simulink model "RobotControl"  (R2016a)
settings: Solver=FixedStepDiscrete  StartTime=0.0  StopTime=16  FixedStep=0.005  RelTol=1e-3
values from neighbouring files (symbols this model uses):
  BACKWARD = 2    [ControlInit.m]
  BUSY = 4    [ControlInit.m]
  CCW = 4    [ControlInit.m]
  CLEANED = 2    [ControlInit.m]
  CW = 3    [ControlInit.m]
  EMPTY = 3    [ControlInit.m]
  FORWARD = 1    [ControlInit.m]
  GTSP = 25    [ControlInit.m]
  initX = uint8((ROOM_SIDE_SIZE/2) - 1)    [ControlInit.m]
  initY = initX    [ControlInit.m]
  LEFT_BUSY_RIGHT_BUSY = 9    [ControlInit.m]
  LEFT_BUSY_RIGHT_CLEANED = 14    [ControlInit.m]
  LEFT_BUSY_RIGHT_EMPTY = 7    [ControlInit.m]
  LEFT_CLEANED_RIGHT_BUSY = 13    [ControlInit.m]
  LEFT_CLEANED_RIGHT_CLEANED = 12    [ControlInit.m]
  LEFT_CLEANED_RIGHT_EMPTY = 10    [ControlInit.m]
  LEFT_EMPTY_RIGHT_BUSY = 8    [ControlInit.m]
  LEFT_EMPTY_RIGHT_CLEANED = 11    [ControlInit.m]
  LEFT_EMPTY_RIGHT_EMPTY = 15    [ControlInit.m]
  map = uint8(ones(ROOM_SIDE_SIZE , ROOM_SIDE_SIZE)*UNCOVERED)    [ControlInit.m]
  MOVE_TURN_LEFT = 20    [ControlInit.m]
  MOVE_TURN_RIGHT = 21    [ControlInit.m]
  MOVE_U_TURN = 24    [ControlInit.m]
  MOVE_U_TURN_LEFT = 23    [ControlInit.m]
  MOVE_U_TURN_RIGHT = 22    [ControlInit.m]
  ROB_EAST = 0    [ControlInit.m]
  ROB_ERRVAL = 5    [ControlInit.m]
  ROB_NONE = 400    [ControlInit.m]
  ROB_NORTH = 270    [ControlInit.m]
  ROB_SOUTH = 90    [ControlInit.m]
  ROB_WEST = 180    [ControlInit.m]
  ROOM_SIDE_SIZE = 20    [ControlInit.m]
  STOP = 5    [ControlInit.m]
  UNCOVERED = 1    [ControlInit.m]
  ZIGZAG = 26    [ControlInit.m]
undefined symbols (not defined in the file or in its folder): COMH, Compass_Handler, MovementHandler, MOVH, POSH, positionHandler, ROB_LENG, ROTH, Routines, SAMPLE_TIME
libraries: simulink x2, SCAN x1, MAPH x1, MOTH x1
(part 1 of 2)
settings Model: Creator=oelkawok  LastModifiedBy=oelkawok
settings DataIOCC: SaveOutput=off  SaveTime=off

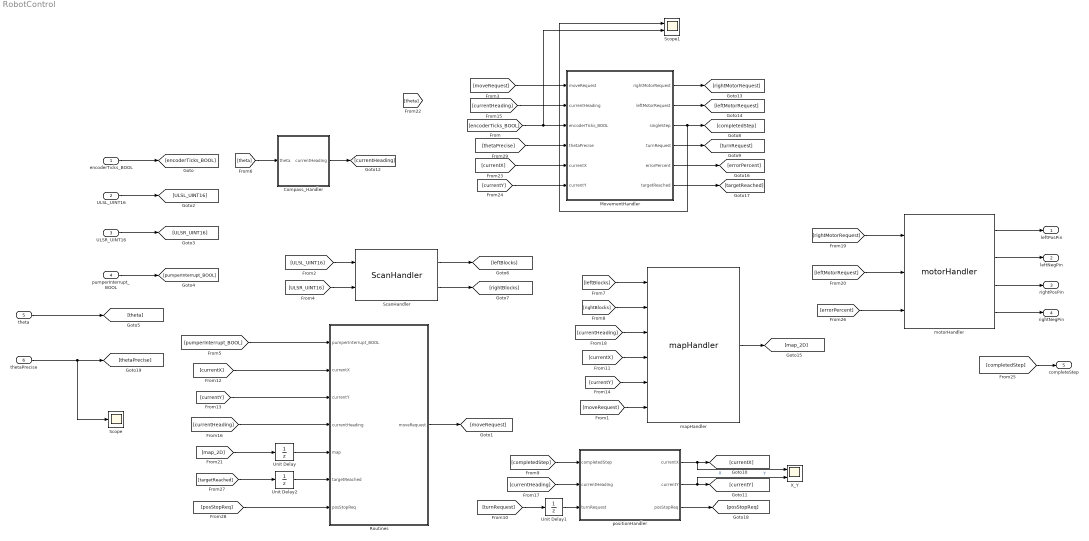
== system RobotControl ==
  encoderTicks_BOOL : Inport  OutDataTypeStr=boolean  PortDimensions=1
  ULSL_UINT16 : Inport  Port=2  PortDimensions=1
  ULSR_UINT16 : Inport  Port=3  PortDimensions=1
  pumperInterrupt_BOOL : Inport  Port=4  OutDataTypeStr=boolean  PortDimensions=1
  theta : Inport  Port=5  OutDataTypeStr=int16  PortDimensions=1
  thetaPrecise : Inport  Port=6  OutDataTypeStr=uint16  PortDimensions=1
  Compass_Handler : Subsystem  AncestorBlock=COMH/Compass_Handler
  MovementHandler : Subsystem  AncestorBlock=MOVH/MovementHandler
  Routines : Subsystem  AncestorBlock=ROTH/Routines
  ScanHandler : SCAN/ScanHandler
  Scope : Scope
  Scope1 : Scope  NumInputPorts=2
  Unit Delay : UnitDelay  InitialCondition=map  SampleTime=-1
      settings: AttributesFormatString=%<InitialCondition>
  Unit Delay1 : UnitDelay  InitialCondition=STOP  SampleTime=-1
      settings: AttributesFormatString=%<InitialCondition>
  Unit Delay2 : UnitDelay  SampleTime=-1
  X_Y : Scope  NumInputPorts=2
  mapHandler : MAPH/mapHandler
  motorHandler : MOTH/motorHandler
  positionHandler : Subsystem  AncestorBlock=POSH/positionHandler
  leftPosPin : Outport  OutDataTypeStr=double  PortDimensions=1
  leftNegPin : Outport  Port=2  OutDataTypeStr=double  PortDimensions=1
  rightPosPin : Outport  Port=3  OutDataTypeStr=double  PortDimensions=1
  rightNegPin : Outport  Port=4  OutDataTypeStr=double  PortDimensions=1
  completeStep : Outport  Port=5  PortDimensions=1
  wires:
  [moveRequest] -> MovementHandler/1(moveRequest)
  [encoderTicks_BOOL] -> MovementHandler/3(encoderTicks_BOOL), Scope1/2
  encoderTicks_BOOL/1 -> [encoderTicks_BOOL]
  ULSL_UINT16/1 -> [ULSL_UINT16]
  [ULSL_UINT16] -> ScanHandler/1
  ULSR_UINT16/1 -> [ULSR_UINT16]
  [ULSR_UINT16] -> ScanHandler/2
  pumperInterrupt_BOOL/1 -> [pumperInterrupt_BOOL]
  [pumperInterrupt_BOOL] -> Routines/1(pumperInterrupt_BOOL)
  Routines/1(moveRequest) -> [moveRequest]
  [moveRequest] -> mapHandler/6
  [theta] -> Compass_Handler/1(theta)
  ScanHandler/1 -> [leftBlocks]
  [leftBlocks] -> mapHandler/1
  ScanHandler/2 -> [rightBlocks]
  [rightBlocks] -> mapHandler/2
  MovementHandler/3(singleStep) -> Scope1/1, [completedStep]
  [completedStep] -> positionHandler/1(completedStep)
  MovementHandler/4(turnRequest) -> [turnRequest]
  [turnRequest] -> Unit Delay1/1
  positionHandler/1(currentX) -> X_Y/1, [currentX]  "X"
  [currentX] -> mapHandler/4
  [currentX] -> Routines/2(currentX)
  positionHandler/2(currentY) -> X_Y/2, [currentY]  "Y"
  [currentY] -> Routines/3(currentY)
  [currentY] -> mapHandler/5
  Compass_Handler/1(currentHeading) -> [currentHeading]
  [currentHeading] -> MovementHandler/2(currentHeading)
  [currentHeading] -> Routines/4(currentHeading)
  [currentHeading] -> positionHandler/2(currentHeading)
  [currentHeading] -> mapHandler/3
  [rightMotorRequest] -> motorHandler/1
  [leftMotorRequest] -> motorHandler/2
  MovementHandler/2(leftMotorRequest) -> [leftMotorRequest]
  MovementHandler/1(rightMotorRequest) -> [rightMotorRequest]
  motorHandler/4 -> rightNegPin/1
  motorHandler/2 -> leftNegPin/1
  motorHandler/3 -> rightPosPin/1
  motorHandler/1 -> leftPosPin/1
  mapHandler/1 -> [map_2D]
  [map_2D] -> Unit Delay/1
  Unit Delay/1 -> Routines/5(map)
  Unit Delay1/1 -> positionHandler/3(turnRequest)
  [currentX] -> MovementHandler/5(currentX)
  [currentY] -> MovementHandler/6(currentY)
  [completedStep] -> completeStep/1
  [errorPercent] -> motorHandler/3
  MovementHandler/5(errorPercent) -> [errorPercent]
  MovementHandler/6(targetReached) -> [targetReached]
  [targetReached] -> Unit Delay2/1
  Unit Delay2/1 -> Routines/6(targetReached)
  positionHandler/3(posStopReq) -> [posStopReq]
  [posStopReq] -> Routines/7(posStopReq)
  theta/1 -> [theta]
  [thetaPrecise] -> MovementHandler/4(thetaPrecise)
  thetaPrecise/1 -> Scope/1, [thetaPrecise]

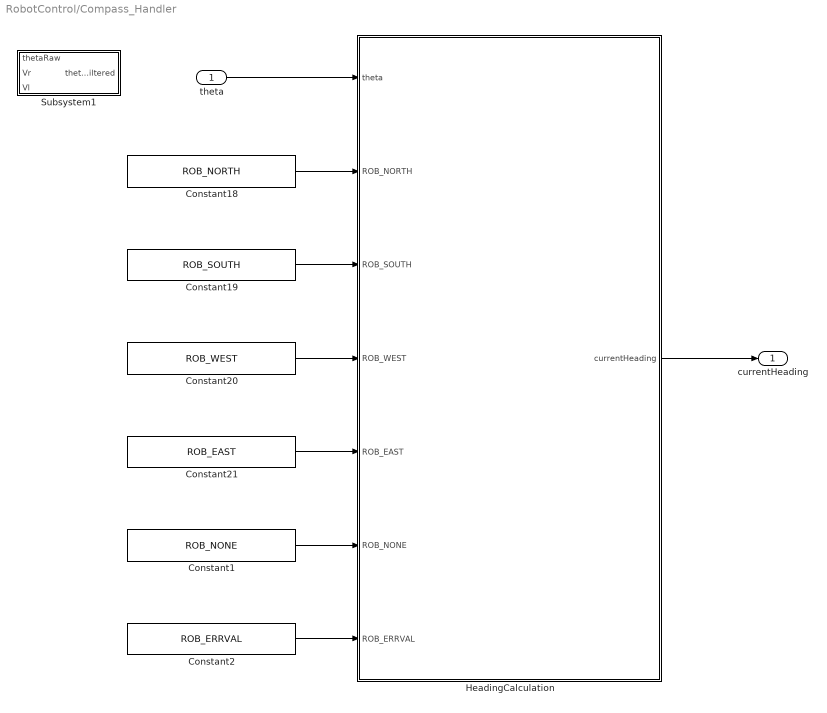
== system RobotControl/Compass_Handler ==
  theta : Inport
  Constant1 : Constant  Value=ROB_NONE
  Constant18 : Constant  Value=ROB_NORTH
  Constant19 : Constant  Value=ROB_SOUTH
  Constant2 : Constant  Value=ROB_ERRVAL
  Constant20 : Constant  Value=ROB_WEST
  Constant21 : Constant  Value=ROB_EAST
  HeadingCalculation : Stateflow chart  TreatAsAtomicUnit=on
  Subsystem1 : Subsystem
  currentHeading : Outport
  wires:
  Constant2/1 -> HeadingCalculation/7(ROB_ERRVAL)
  Constant1/1 -> HeadingCalculation/6(ROB_NONE)
  Constant21/1 -> HeadingCalculation/5(ROB_EAST)
  Constant20/1 -> HeadingCalculation/4(ROB_WEST)
  Constant19/1 -> HeadingCalculation/3(ROB_SOUTH)
  Constant18/1 -> HeadingCalculation/2(ROB_NORTH)
  theta/1 -> HeadingCalculation/1(theta)
  HeadingCalculation/1(currentHeading) -> currentHeading/1

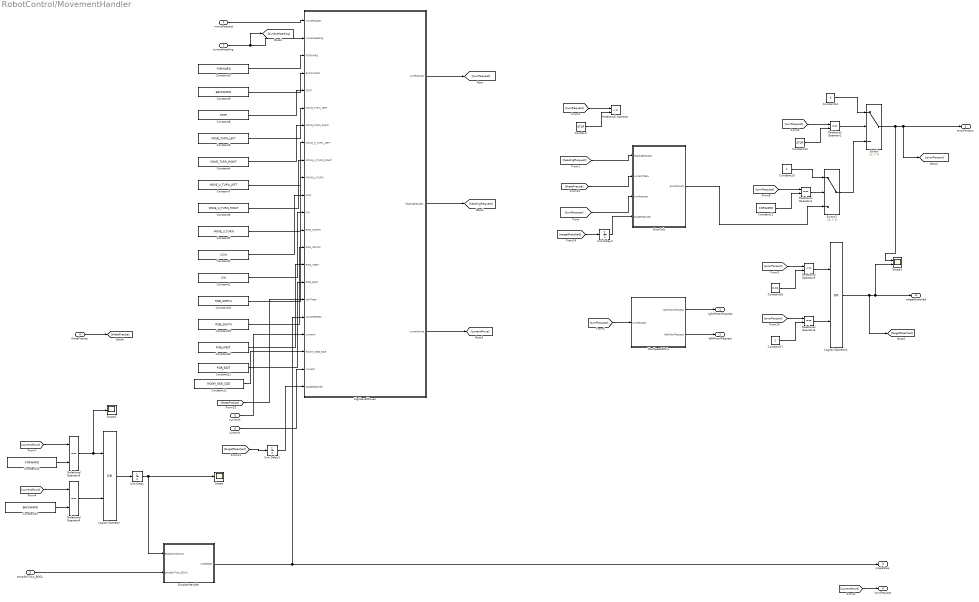
== system RobotControl/MovementHandler ==
  moveRequest : Inport
  currentHeading : Inport  Port=2
  encoderTicks_BOOL : Inport  Port=3  PortDimensions=1
  thetaPrecise : Inport  Port=4  PortDimensions=1
  currentX : Inport  Port=5  PortDimensions=1
  currentY : Inport  Port=6  PortDimensions=1
  Constant : Constant  Value=STOP
  Constant1 : Constant  Value=CW
  Constant10 : Constant  Value=FORWARD
  Constant11 : Constant  Value=ROOM_SIDE_SIZE
  Constant12 : Constant  Value=FORWARD
  Constant13 : Constant  Value=STOP
  Constant14 : Constant  Value=0
  Constant15 : Constant
  Constant16 : Constant  Value=0.01
  Constant17 : Constant
  Constant18 : Constant  Value=ROB_NORTH
  Constant19 : Constant  Value=ROB_SOUTH
  Constant2 : Constant  Value=CCW
  Constant20 : Constant  Value=ROB_WEST
  Constant21 : Constant  Value=ROB_EAST
  Constant29 : Constant  Value=BACKWARD
  Constant3 : Constant  Value=MOVE_TURN_LEFT
  Constant30 : Constant  Value=FORWARD
  Constant4 : Constant  Value=MOVE_TURN_RIGHT
  Constant5 : Constant  Value=MOVE_U_TURN
  Constant6 : Constant  Value=MOVE_U_TURN_RIGHT
  Constant7 : Constant  Value=MOVE_U_TURN_LEFT
  Constant8 : Constant  Value=STOP
  Constant9 : Constant  Value=BACKWARD
  EncoderHandler : Subsystem
  ErrorCalc : Subsystem
  HighLevelMoves : Stateflow chart  TreatAsAtomicUnit=on
  Logical Operator : Logic  Operator=OR  AllPortsSameDT=off  OutDataTypeStr=boolean
  Logical Operator1 : Logic  Operator=OR  AllPortsSameDT=off  OutDataTypeStr=boolean
  MaxSpeedsOnly : Subsystem
  Relational Operator : RelationalOperator  Operator=~=  OutDataTypeStr=boolean
  Relational Operator{1..2,4..6} (5 alike) : RelationalOperator  Operator===  OutDataTypeStr=boolean
  Relational Operator3 : RelationalOperator  Operator=<=  OutDataTypeStr=boolean
  Scope : Scope
  Scope1 : Scope
  Scope2 : Scope  NumInputPorts=2
  Switch : Switch  Criteria=u2 > Threshold
  Switch1 : Switch  Criteria=u2 > Threshold
  Unit Delay : UnitDelay  SampleTime=-1
  Unit Delay1 : UnitDelay  SampleTime=-1
  Unit Delay2 : UnitDelay  SampleTime=-1
  rightMotorRequest : Outport
  leftMotorRequest : Outport  Port=2
  singleStep : Outport  Port=3
  turnRequest : Outport  Port=4
  errorPercent : Outport  Port=5  OutputWhenDisabled=reset  InitialOutput=0
  targetReached : Outport  Port=6  OutputWhenDisabled=reset  InitialOutput=0
  wires:
  MaxSpeedsOnly/1(rightMotorRequest) -> rightMotorRequest/1
  MaxSpeedsOnly/2(leftMotorRequest) -> leftMotorRequest/1
  [turnRequest] -> MaxSpeedsOnly/1(turnRequest)
  Constant/1 -> Relational Operator/2
  [turnRequest] -> Relational Operator/1
  HighLevelMoves/3(currentMove) -> [currentMove]
  [headingRequest] -> ErrorCalc/1(headingRequest)
  [thetaPrecise] -> ErrorCalc/2(currentTheta)
  [turnRequest] -> ErrorCalc/3(turnRequest)
  [currentMove] -> turnRequest/1
  EncoderHandler/1(singleStep) -> HighLevelMoves/18(completeStep), singleStep/1
  Logical Operator/1 -> Unit Delay/1
  Relational Operator4/1 -> Logical Operator/2
  Relational Operator5/1 -> Scope1/1, Logical Operator/1
  [currentMove] -> Relational Operator5/1
  Constant30/1 -> Relational Operator5/2
  [currentMove] -> Relational Operator4/1
  Constant29/1 -> Relational Operator4/2
  HighLevelMoves/1(turnRequest) -> [turnRequest]
  Constant8/1 -> HighLevelMoves/5(STOP)
  Constant9/1 -> HighLevelMoves/4(BACKWARD)
  Constant10/1 -> HighLevelMoves/3(FORWARD)
  Constant7/1 -> HighLevelMoves/8(MOVE_U_TURN_LEFT)
  Constant6/1 -> HighLevelMoves/9(MOVE_U_TURN_RIGHT)
  Constant4/1 -> HighLevelMoves/7(MOVE_TURN_RIGHT)
  Constant3/1 -> HighLevelMoves/6(MOVE_TURN_LEFT)
  Constant5/1 -> HighLevelMoves/10(MOVE_U_TURN)
  Constant2/1 -> HighLevelMoves/11(CCW)
  Constant1/1 -> HighLevelMoves/12(CW)
  Constant21/1 -> HighLevelMoves/16(ROB_EAST)
  Constant20/1 -> HighLevelMoves/15(ROB_WEST)
  Constant19/1 -> HighLevelMoves/14(ROB_SOUTH)
  Constant18/1 -> HighLevelMoves/13(ROB_NORTH)
  encoderTicks_BOOL/1 -> EncoderHandler/2(encoderTicks_BOOL)
  currentHeading/1 -> [currentHeading], HighLevelMoves/2(currentHeading)
  moveRequest/1 -> HighLevelMoves/1(moveRequest)
  HighLevelMoves/2(headingRequest) -> [headingRequest]
  Unit Delay/1 -> Scope/1, EncoderHandler/1(EnableConditions)
  currentX/1 -> HighLevelMoves/19(currentX)
  currentY/1 -> HighLevelMoves/21(currentY)
  Constant11/1 -> HighLevelMoves/20(ROOM_SIDE_SIZE)
  Constant13/1 -> Relational Operator2/2
  [turnRequest] -> Relational Operator2/1
  Relational Operator2/1 -> Switch/2
  Constant14/1 -> Switch/1
  Switch1/1 -> Switch/3
  Constant12/1 -> Relational Operator1/2
  [turnRequest] -> Relational Operator1/1
  Relational Operator1/1 -> Switch1/2
  Constant15/1 -> Switch1/1
  ErrorCalc/1(errorPercent) -> Switch1/3
  Switch/1 -> Scope2/1, [errorPercent], errorPercent/1
  [errorPercent] -> Relational Operator3/1
  Constant16/1 -> Relational Operator3/2
  [errorPercent] -> Relational Operator6/1
  Constant17/1 -> Relational Operator6/2
  Relational Operator3/1 -> Logical Operator1/1
  Relational Operator6/1 -> Logical Operator1/2
  Logical Operator1/1 -> [targetReached], Scope2/2, targetReached/1
  [targetReached] -> Unit Delay1/1
  Unit Delay1/1 -> HighLevelMoves/22(targetReached)
  thetaPrecise/1 -> [thetaPrecise]
  [thetaPrecise] -> HighLevelMoves/17(rawTheta)
  [targetReached] -> Unit Delay2/1
  Unit Delay2/1 -> ErrorCalc/4(targetReached)

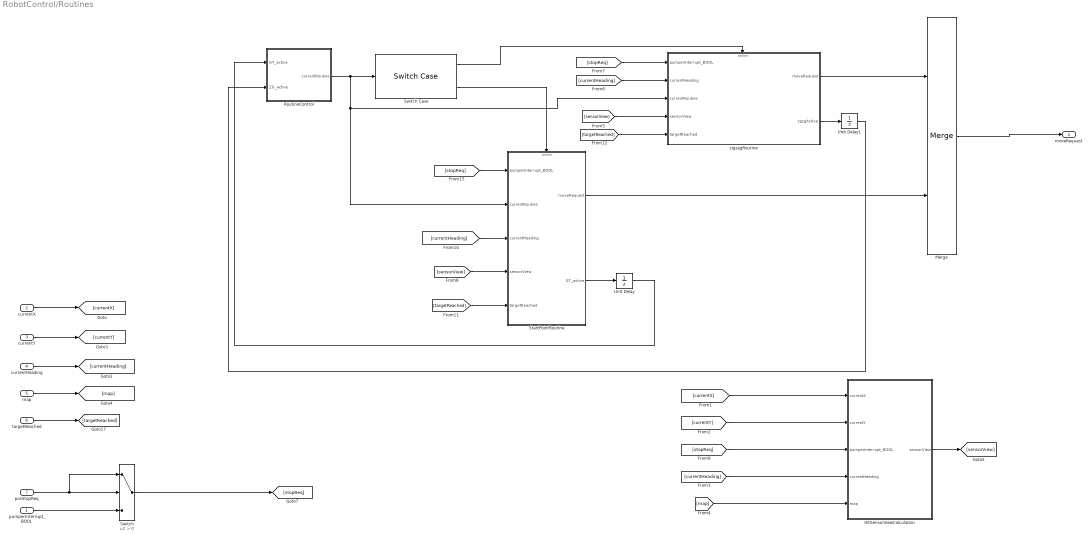
== system RobotControl/Routines ==
  pumperInterrupt_BOOL : Inport
  currentX : Inport  Port=2
  currentY : Inport  Port=3
  currentHeading : Inport  Port=4
  map : Inport  Port=5
  targetReached : Inport  Port=6
  posStopReq : Inport  Port=7
  HitSensorViewCalculation : Subsystem
  Merge : Merge  InitialOutput=5
      settings: AttributesFormatString=%<InitialOutput>
  RoutineControl : Subsystem
  StartPointRoutine : Subsystem
  Switch : Switch  Criteria=u2 > Threshold
  Switch Case : SwitchCase  CaseConditions={ZIGZAG, GTSP}  ShowDefaultCase=off
      settings: AttributesFormatString=%<CaseConditions>
  Unit Delay : UnitDelay  InitialCondition=true  SampleTime=-1
  Unit Delay1 : UnitDelay  InitialCondition=false  SampleTime=-1
  zigzagRoutine : Subsystem
  moveRequest : Outport
  wires:
  map/1 -> [map]
  currentX/1 -> [currentX]
  currentY/1 -> [currentY]
  currentHeading/1 -> [currentHeading]
  Unit Delay/1 -> RoutineControl/1(GT_active)
  StartPointRoutine/2(GT_active) -> Unit Delay/1
  Merge/1 -> moveRequest/1
  HitSensorViewCalculation/1(sensorView) -> [sensorView]
  [sensorView] -> zigzagRoutine/4(sensorView)
  [stopReq] -> zigzagRoutine/1(pumperInterrupt_BOOL)
  [currentHeading] -> zigzagRoutine/2(currentHeading)
  RoutineControl/1(currentRoutine) -> zigzagRoutine/3(currentRoutine), StartPointRoutine/2(currentRoutine), Switch Case/1
  Switch Case/1 -> zigzagRoutine/Action
  Switch Case/2 -> StartPointRoutine/Action
  [map] -> HitSensorViewCalculation/5(map)
  [currentHeading] -> HitSensorViewCalculation/4(currentHeading)
  [stopReq] -> HitSensorViewCalculation/3(pumperInterrupt_BOOL)
  [currentY] -> HitSensorViewCalculation/2(currentY)
  [currentX] -> HitSensorViewCalculation/1(currentX)
  StartPointRoutine/1(moveRequest) -> Merge/2
  zigzagRoutine/1(moveRequest) -> Merge/1
  zigzagRoutine/2(zgzgActive) -> Unit Delay1/1
  Unit Delay1/1 -> RoutineControl/2(ZG_active)
  [stopReq] -> StartPointRoutine/1(pumperInterrupt_BOOL)
  [sensorView] -> StartPointRoutine/4(sensorView)
  [currentHeading] -> StartPointRoutine/3(currentHeading)
  targetReached/1 -> [targetReached]
  [targetReached] -> StartPointRoutine/5(targetReached)
  [targetReached] -> zigzagRoutine/5(targetReached)
  posStopReq/1 -> Switch/1, Switch/2
  Switch/1 -> [stopReq]
  pumperInterrupt_BOOL/1 -> Switch/3

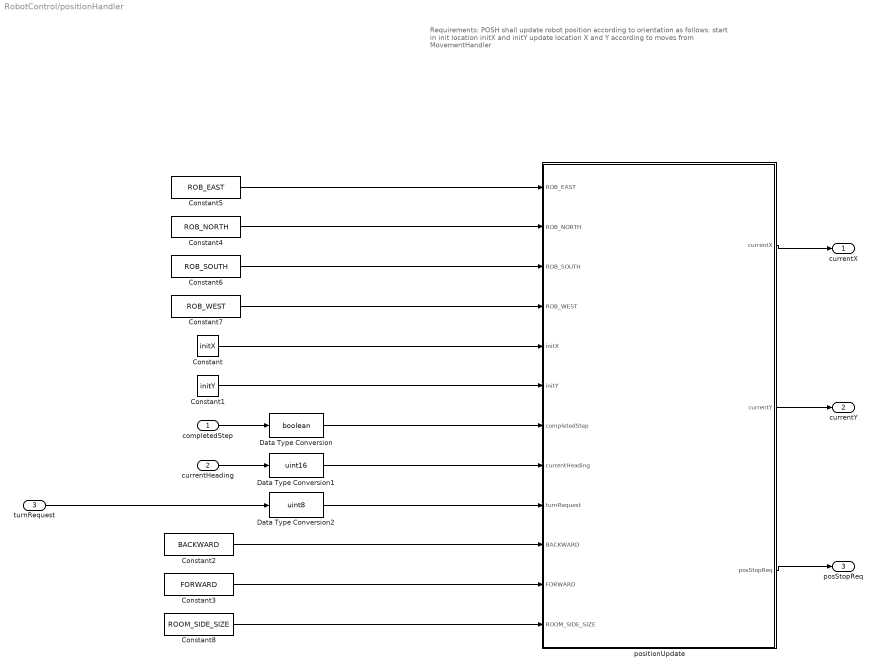
== system RobotControl/positionHandler ==
  note: Requirements:
      | POSH shall update robot position according to orientation as follows:
      | start in init location initX and initY
      | update location X and Y according to moves from MovementHandler
  completedStep : Inport
  currentHeading : Inport  Port=2
  turnRequest : Inport  Port=3
  Constant : Constant  Value=initX
  Constant1 : Constant  Value=initY
  Constant2 : Constant  Value=BACKWARD
  Constant3 : Constant  Value=FORWARD
  Constant4 : Constant  Value=ROB_NORTH
  Constant5 : Constant  Value=ROB_EAST
  Constant6 : Constant  Value=ROB_SOUTH
  Constant7 : Constant  Value=ROB_WEST
  Constant8 : Constant  Value=ROOM_SIDE_SIZE
  Data Type Conversion : DataTypeConversion  OutDataTypeStr=boolean
  Data Type Conversion1 : DataTypeConversion  OutDataTypeStr=uint16
  Data Type Conversion2 : DataTypeConversion  OutDataTypeStr=uint8
  positionUpdate : Stateflow chart  TreatAsAtomicUnit=on
  currentX : Outport
  currentY : Outport  Port=2
  posStopReq : Outport  Port=3
  wires:
  Constant/1 -> positionUpdate/5(initX)
  Constant1/1 -> positionUpdate/6(initY)
  Constant6/1 -> positionUpdate/3(ROB_SOUTH)
  Constant7/1 -> positionUpdate/4(ROB_WEST)
  Constant4/1 -> positionUpdate/2(ROB_NORTH)
  Constant5/1 -> positionUpdate/1(ROB_EAST)
  positionUpdate/2(currentY) -> currentY/1
  positionUpdate/1(currentX) -> currentX/1
  currentHeading/1 -> Data Type Conversion1/1
  completedStep/1 -> Data Type Conversion/1
  turnRequest/1 -> Data Type Conversion2/1
  Data Type Conversion/1 -> positionUpdate/7(completedStep)
  Data Type Conversion1/1 -> positionUpdate/8(currentHeading)
  Data Type Conversion2/1 -> positionUpdate/9(turnRequest)
  Constant3/1 -> positionUpdate/11(FORWARD)
  Constant2/1 -> positionUpdate/10(BACKWARD)
  positionUpdate/3(posStopReq) -> posStopReq/1
  Constant8/1 -> positionUpdate/12(ROOM_SIDE_SIZE)

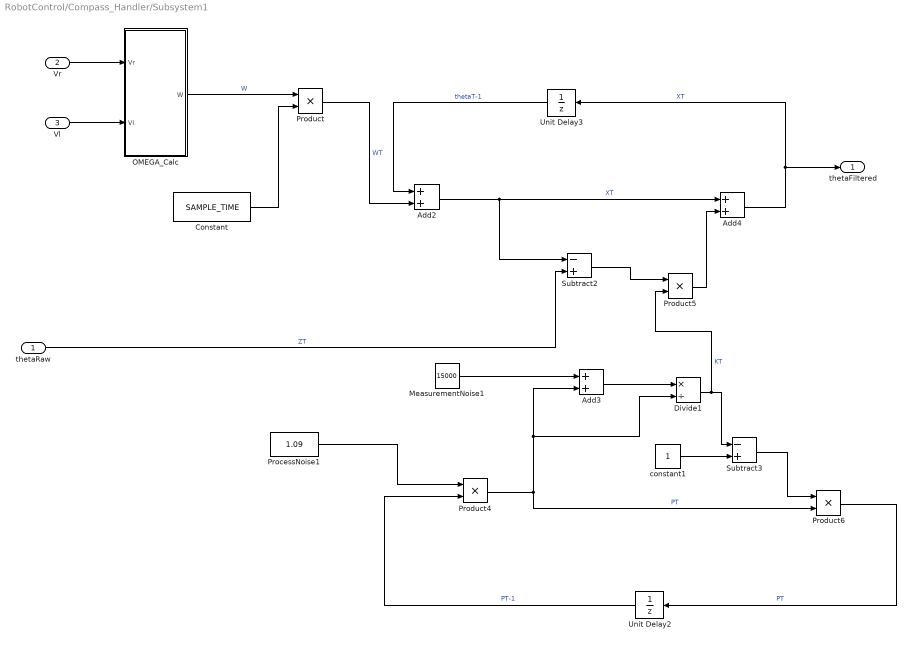
== system RobotControl/Compass_Handler/Subsystem1 ==
  thetaRaw : Inport
  Vr : Inport  Port=2
  Vl : Inport  Port=3
  Add2 : Sum
  Add3 : Sum
  Add4 : Sum
  Constant : Constant  Value=SAMPLE_TIME
  Divide1 : Product  Inputs=*/
  MeasurementNoise1 : Constant  Value=15000
  OMEGA_Calc : Subsystem
  ProcessNoise1 : Constant  Value=1.09
  Product{,4..6} (4 alike) : Product
  Subtract2 : Sum  Inputs=-+
  Subtract3 : Sum  Inputs=-+
  Unit Delay2 : UnitDelay  InitialCondition=1  SampleTime=-1
  Unit Delay3 : UnitDelay  InitialCondition=ROB_NORTH*100  SampleTime=-1
  constant1 : Constant
  thetaFiltered : Outport
  wires:
  Vl/1 -> OMEGA_Calc/2(Vl)
  Vr/1 -> OMEGA_Calc/1(Vr)
  Constant/1 -> Product/2
  OMEGA_Calc/1(W) -> Product/1  "W"
  thetaRaw/1 -> Subtract2/2  "ZT"
  Product/1 -> Add2/2  "WT"
  Unit Delay3/1 -> Add2/1  "thetaT-1"
  ProcessNoise1/1 -> Product4/1
  Unit Delay2/1 -> Product4/2  "PT-1"
  Product4/1 -> Product6/2, Divide1/2, Add3/2  "PT"
  MeasurementNoise1/1 -> Add3/1
  Add3/1 -> Divide1/1
  Divide1/1 -> Subtract3/1, Product5/2  "KT"
  Add2/1 -> Subtract2/1, Add4/1  "XT"
  Subtract2/1 -> Product5/1
  constant1/1 -> Subtract3/2
  Subtract3/1 -> Product6/1
  Product6/1 -> Unit Delay2/1  "PT"
  Product5/1 -> Add4/2
  Add4/1 -> thetaFiltered/1, Unit Delay3/1  "XT"

== system RobotControl/MovementHandler/EncoderHandler ==
  EnableConditions : Inport  PortDimensions=1
  encoderTicks_BOOL : Inport  Port=2  PortDimensions=1
  Unit Delay : UnitDelay  SampleTime=-1
  singleStepCalc : Stateflow chart  TreatAsAtomicUnit=on
  singleStep : Outport  OutputWhenDisabled=reset  InitialOutput=0
      settings: AttributesFormatString=%<OutputWhenDisabled>
  wires:
  singleStepCalc/1(step) -> Unit Delay/1, singleStep/1
  encoderTicks_BOOL/1 -> singleStepCalc/1(encoderTicks_BOOL)
  Unit Delay/1 -> singleStepCalc/3(stepOld)
  EnableConditions/1 -> singleStepCalc/2(EnableConditions)

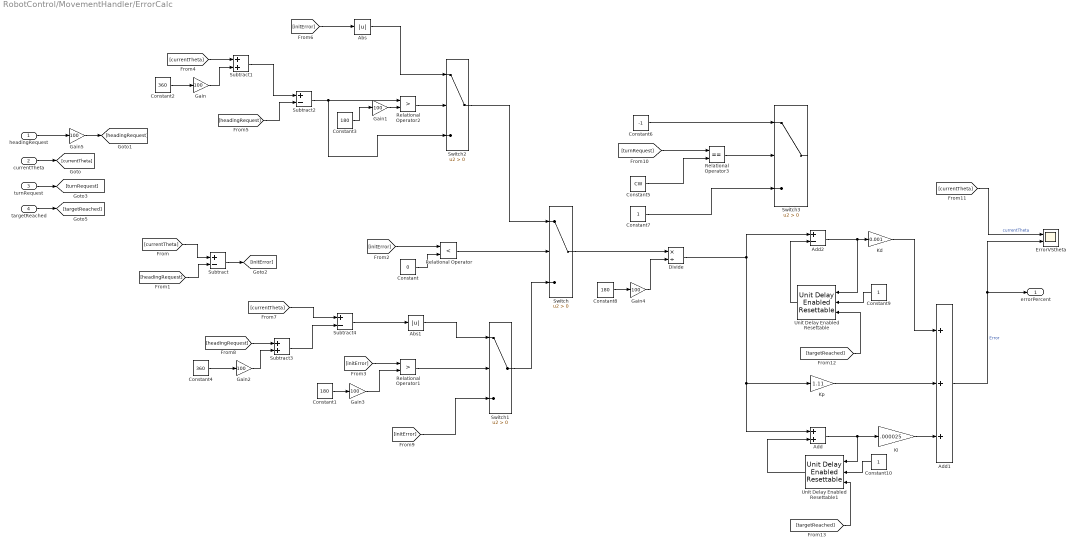
== system RobotControl/MovementHandler/ErrorCalc ==
  headingRequest : Inport
  currentTheta : Inport  Port=2
  turnRequest : Inport  Port=3
  targetReached : Inport  Port=4
  Abs : Abs
  Abs1 : Abs
  Add : Sum
  Add1 : Sum  Inputs=+++
  Add2 : Sum  Inputs=+-
  Constant : Constant  Value=0
  Constant1 : Constant  Value=180
  Constant10 : Constant
  Constant2 : Constant  Value=360
  Constant3 : Constant  Value=180
  Constant4 : Constant  Value=360
  Constant5 : Constant  Value=CW
  Constant6 : Constant  Value=-1
  Constant7 : Constant
  Constant8 : Constant  Value=180
  Constant9 : Constant
  Divide : Product  Inputs=*/
  ErrorVStheta : Scope  NumInputPorts=2
  Gain{,1..5} (6 alike) : Gain  Gain=100
  Kd : Gain  Gain=0.001
  Ki : Gain  Gain=.000025
  Kp : Gain  Gain=1.11
  Relational Operator : RelationalOperator  Operator=<  OutDataTypeStr=boolean
  Relational Operator1 : RelationalOperator  Operator=>  OutDataTypeStr=boolean
  Relational Operator2 : RelationalOperator  Operator=>  OutDataTypeStr=boolean
  Relational Operator3 : RelationalOperator  Operator===  OutDataTypeStr=boolean
  Subtract : Sum  Inputs=+-
  Subtract1 : Sum
  Subtract2 : Sum  Inputs=+-
  Subtract3 : Sum
  Subtract4 : Sum  Inputs=+-
  Switch{,1..3} (4 alike) : Switch  Criteria=u2 > Threshold
  Unit Delay Enabled Resettable : simulink/Additional Math & Discrete/Additional Discrete/Unit Delay Enabled Resettable  vinit=0.0  tsamp=-1
  Unit Delay Enabled Resettable1 : simulink/Additional Math & Discrete/Additional Discrete/Unit Delay Enabled Resettable  vinit=0.0  tsamp=-1
  errorPercent : Outport  OutputWhenDisabled=reset  InitialOutput=0
  wires:
  Constant8/1 -> Gain4/1
  Switch/1 -> Divide/1
  Constant7/1 -> Switch3/3
  Constant6/1 -> Switch3/1
  Relational Operator3/1 -> Switch3/2
  Constant5/1 -> Relational Operator3/2
  [turnRequest] -> Relational Operator3/1
  turnRequest/1 -> [turnRequest]
  [initError] -> Switch1/3
  Abs1/1 -> Switch1/1
  Subtract4/1 -> Abs1/1
  Subtract3/1 -> Subtract4/2
  [currentTheta] -> Subtract4/1
  [headingRequest] -> Subtract3/1
  Constant4/1 -> Gain2/1
  Abs/1 -> Switch2/1
  [initError] -> Abs/1
  Switch2/1 -> Switch/1
  Relational Operator2/1 -> Switch2/2
  Subtract2/1 -> Switch2/3, Relational Operator2/1
  Constant3/1 -> Gain1/1
  [headingRequest] -> Subtract2/2
  Subtract1/1 -> Subtract2/1
  Constant2/1 -> Gain/1
  [currentTheta] -> Subtract1/1
  [initError] -> Relational Operator1/1
  [initError] -> Relational Operator/1
  Subtract/1 -> [initError]
  [currentTheta] -> Subtract/1
  [headingRequest] -> Subtract/2
  currentTheta/1 -> [currentTheta]
  headingRequest/1 -> Gain5/1
  Switch1/1 -> Switch/3
  Constant1/1 -> Gain3/1
  Relational Operator1/1 -> Switch1/2
  Relational Operator/1 -> Switch/2
  Constant/1 -> Relational Operator/2
  Divide/1 -> Add2/1, Kp/1, Add/1
  Add/1 -> Unit Delay Enabled Resettable1/1, Ki/1
  Unit Delay Enabled Resettable1/1 -> Add/2
  Ki/1 -> Add1/3
  Add2/1 -> Unit Delay Enabled Resettable/1, Kd/1
  Unit Delay Enabled Resettable/1 -> Add2/2
  Kd/1 -> Add1/1
  Kp/1 -> Add1/2
  Add1/1 -> ErrorVStheta/2, errorPercent/1  "Error"
  [currentTheta] -> ErrorVStheta/1  "currentTheta"
  Gain/1 -> Subtract1/2
  Gain1/1 -> Relational Operator2/2
  Gain2/1 -> Subtract3/2
  Gain3/1 -> Relational Operator1/2
  Gain4/1 -> Divide/2
  Gain5/1 -> [headingRequest]
  Constant9/1 -> Unit Delay Enabled Resettable/2
  targetReached/1 -> [targetReached]
  [targetReached] -> Unit Delay Enabled Resettable/3
  Constant10/1 -> Unit Delay Enabled Resettable1/2
  [targetReached] -> Unit Delay Enabled Resettable1/3

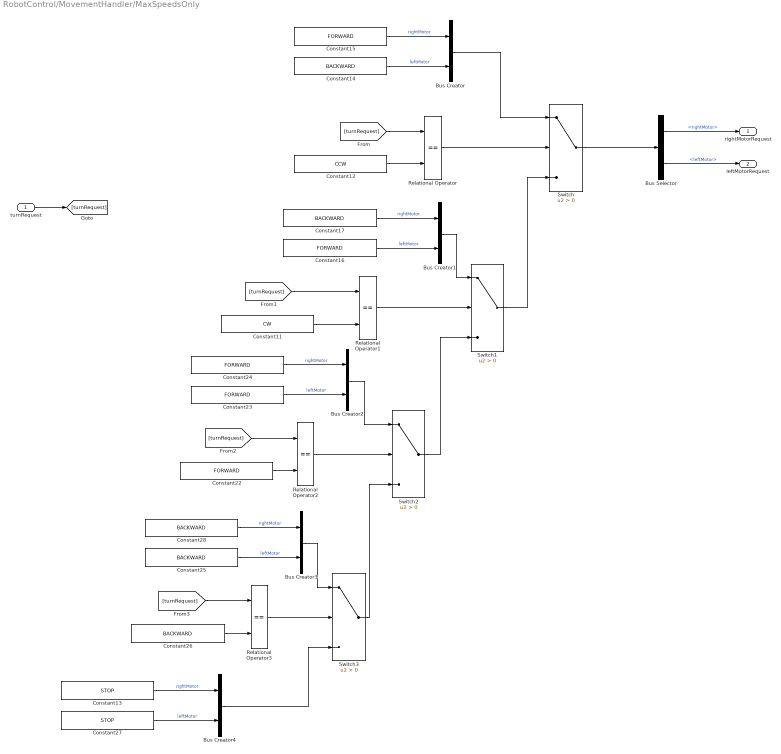
== system RobotControl/MovementHandler/MaxSpeedsOnly ==
  turnRequest : Inport
  Bus Creator{,1..4} (5 alike) : BusCreator  Inputs=2
  Bus Selector : BusSelector  OutputSignals=rightMotor,leftMotor
  Constant11 : Constant  Value=CW
  Constant12 : Constant  Value=CCW
  Constant13 : Constant  Value=STOP
  Constant{14,17,25..26,28} (5 alike) : Constant  Value=BACKWARD
  Constant{15..16,22..24} (5 alike) : Constant  Value=FORWARD
  Constant27 : Constant  Value=STOP
  Relational Operator{,1..3} (4 alike) : RelationalOperator  Operator===  OutDataTypeStr=boolean
  Switch{,1..3} (4 alike) : Switch  Criteria=u2 > Threshold
  rightMotorRequest : Outport
  leftMotorRequest : Outport  Port=2
  wires:
  Constant15/1 -> Bus Creator/1  "rightMotor"
  Constant12/1 -> Relational Operator/2
  Relational Operator/1 -> Switch/2
  [turnRequest] -> Relational Operator/1
  Switch/1 -> Bus Selector/1
  Constant14/1 -> Bus Creator/2  "leftMotor"
  Bus Creator/1 -> Switch/1
  [turnRequest] -> Relational Operator1/1
  Bus Selector/1 -> rightMotorRequest/1  "<rightMotor>"
  Constant16/1 -> Bus Creator1/2  "leftMotor"
  Bus Selector/2 -> leftMotorRequest/1  "<leftMotor>"
  Switch1/1 -> Switch/3
  [turnRequest] -> Relational Operator3/1
  Constant17/1 -> Bus Creator1/1  "rightMotor"
  Bus Creator1/1 -> Switch1/1
  Constant11/1 -> Relational Operator1/2
  Constant24/1 -> Bus Creator2/1  "rightMotor"
  Relational Operator1/1 -> Switch1/2
  Relational Operator3/1 -> Switch3/2
  [turnRequest] -> Relational Operator2/1
  Constant22/1 -> Relational Operator2/2
  Switch2/1 -> Switch1/3
  Relational Operator2/1 -> Switch2/2
  Constant28/1 -> Bus Creator3/1  "rightMotor"
  Constant25/1 -> Bus Creator3/2  "leftMotor"
  Constant26/1 -> Relational Operator3/2
  Bus Creator2/1 -> Switch2/1
  Bus Creator4/1 -> Switch3/3
  Switch3/1 -> Switch2/3
  Constant27/1 -> Bus Creator4/2  "leftMotor"
  Bus Creator3/1 -> Switch3/1
  Constant23/1 -> Bus Creator2/2  "leftMotor"
  Constant13/1 -> Bus Creator4/1  "rightMotor"
  turnRequest/1 -> [turnRequest]

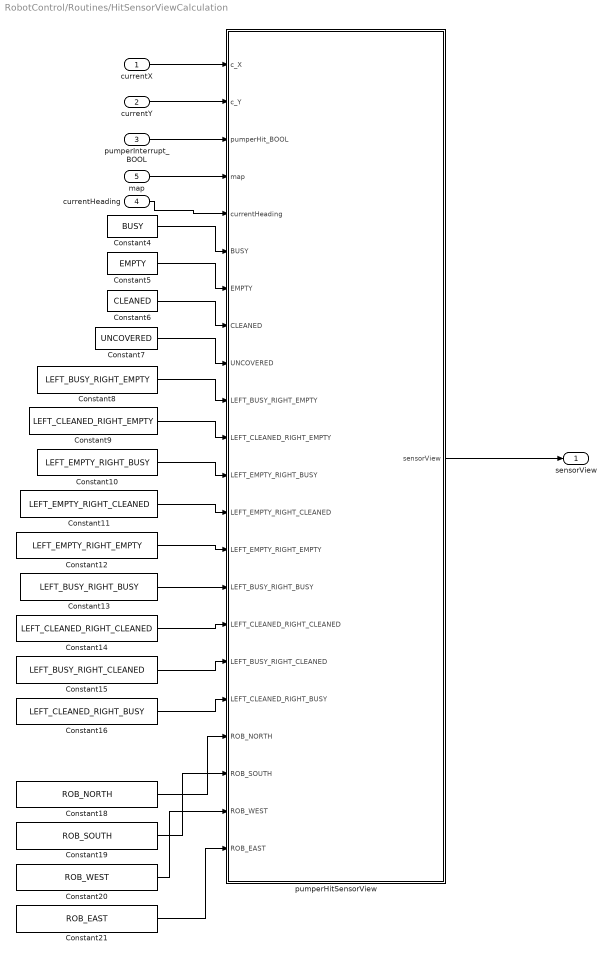
== system RobotControl/Routines/HitSensorViewCalculation ==
  currentX : Inport
  currentY : Inport  Port=2
  pumperInterrupt_BOOL : Inport  Port=3
  currentHeading : Inport  Port=4
  map : Inport  Port=5
  Constant10 : Constant  Value=LEFT_EMPTY_RIGHT_BUSY
  Constant11 : Constant  Value=LEFT_EMPTY_RIGHT_CLEANED
  Constant12 : Constant  Value=LEFT_EMPTY_RIGHT_EMPTY
  Constant13 : Constant  Value=LEFT_BUSY_RIGHT_BUSY
  Constant14 : Constant  Value=LEFT_CLEANED_RIGHT_CLEANED
  Constant15 : Constant  Value=LEFT_BUSY_RIGHT_CLEANED
  Constant16 : Constant  Value=LEFT_CLEANED_RIGHT_BUSY
  Constant18 : Constant  Value=ROB_NORTH
  Constant19 : Constant  Value=ROB_SOUTH
  Constant20 : Constant  Value=ROB_WEST
  Constant21 : Constant  Value=ROB_EAST
  Constant4 : Constant  Value=BUSY
  Constant5 : Constant  Value=EMPTY
  Constant6 : Constant  Value=CLEANED
  Constant7 : Constant  Value=UNCOVERED
  Constant8 : Constant  Value=LEFT_BUSY_RIGHT_EMPTY
  Constant9 : Constant  Value=LEFT_CLEANED_RIGHT_EMPTY
  pumperHitSensorView : Stateflow chart  TreatAsAtomicUnit=on
  sensorView : Outport
  wires:
  currentHeading/1 -> pumperHitSensorView/5(currentHeading)
  pumperHitSensorView/1(sensorView) -> sensorView/1
  Constant16/1 -> pumperHitSensorView/18(LEFT_CLEANED_RIGHT_BUSY)
  Constant14/1 -> pumperHitSensorView/16(LEFT_CLEANED_RIGHT_CLEANED)
  Constant11/1 -> pumperHitSensorView/13(LEFT_EMPTY_RIGHT_CLEANED)
  Constant9/1 -> pumperHitSensorView/11(LEFT_CLEANED_RIGHT_EMPTY)
  Constant13/1 -> pumperHitSensorView/15(LEFT_BUSY_RIGHT_BUSY)
  Constant12/1 -> pumperHitSensorView/14(LEFT_EMPTY_RIGHT_EMPTY)
  Constant15/1 -> pumperHitSensorView/17(LEFT_BUSY_RIGHT_CLEANED)
  Constant10/1 -> pumperHitSensorView/12(LEFT_EMPTY_RIGHT_BUSY)
  Constant6/1 -> pumperHitSensorView/8(CLEANED)
  Constant4/1 -> pumperHitSensorView/6(BUSY)
  Constant5/1 -> pumperHitSensorView/7(EMPTY)
  Constant7/1 -> pumperHitSensorView/9(UNCOVERED)
  Constant8/1 -> pumperHitSensorView/10(LEFT_BUSY_RIGHT_EMPTY)
  currentY/1 -> pumperHitSensorView/2(c_Y)
  currentX/1 -> pumperHitSensorView/1(c_X)
  pumperInterrupt_BOOL/1 -> pumperHitSensorView/3(pumperHit_BOOL)
  map/1 -> pumperHitSensorView/4(map)
  Constant20/1 -> pumperHitSensorView/21(ROB_WEST)
  Constant18/1 -> pumperHitSensorView/19(ROB_NORTH)
  Constant21/1 -> pumperHitSensorView/22(ROB_EAST)
  Constant19/1 -> pumperHitSensorView/20(ROB_SOUTH)

== system RobotControl/Routines/RoutineControl ==
  GT_active : Inport
  ZG_active : Inport  Port=2
  Chart : Stateflow chart  TreatAsAtomicUnit=on
  Constant : Constant  Value=GTSP
  Constant1 : Constant  Value=ZIGZAG
  currentRoutine : Outport
  wires:
  Constant1/1 -> Chart/4(ZIGZAG)
  Constant/1 -> Chart/3(GTSP)
  Chart/1(currentRoutine) -> currentRoutine/1
  GT_active/1 -> Chart/1(GT_active)
  ZG_active/1 -> Chart/2(ZG_active)

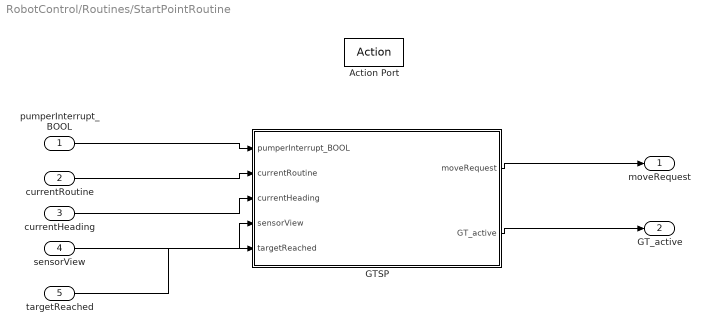
== system RobotControl/Routines/StartPointRoutine ==
  pumperInterrupt_BOOL : Inport
  currentRoutine : Inport  Port=2
  currentHeading : Inport  Port=3
  sensorView : Inport  Port=4
  targetReached : Inport  Port=5
  Action Port : ActionPort  ActionType=case
  GTSP : Subsystem
  moveRequest : Outport
  GT_active : Outport  Port=2  InitialOutput=true
  wires:
  GTSP/2(GT_active) -> GT_active/1
  GTSP/1(moveRequest) -> moveRequest/1
  currentHeading/1 -> GTSP/3(currentHeading)
  currentRoutine/1 -> GTSP/2(currentRoutine)
  pumperInterrupt_BOOL/1 -> GTSP/1(pumperInterrupt_BOOL)
  sensorView/1 -> GTSP/4(sensorView)
  targetReached/1 -> GTSP/5(targetReached)

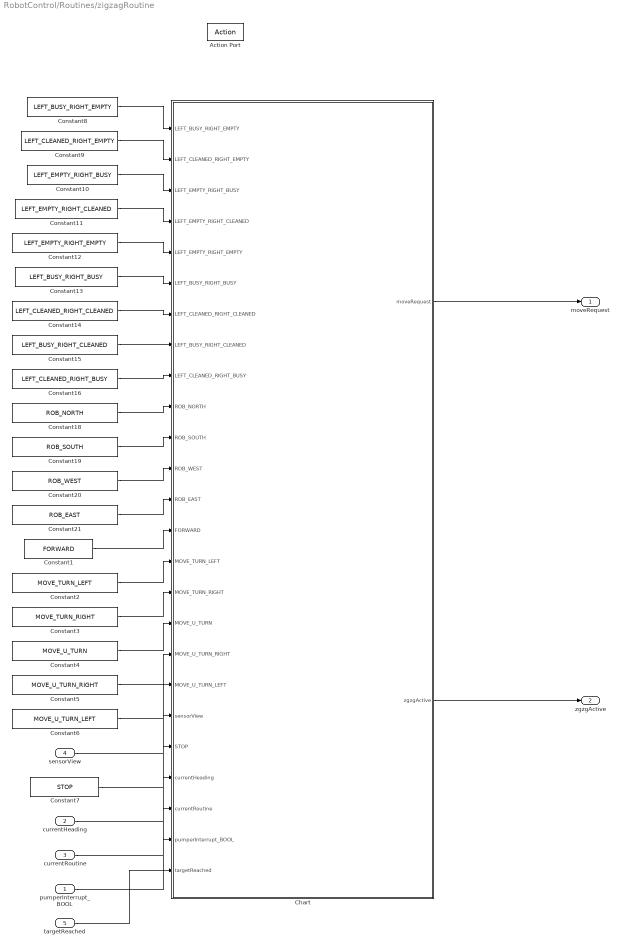
== system RobotControl/Routines/zigzagRoutine ==
  pumperInterrupt_BOOL : Inport
  currentHeading : Inport  Port=2
  currentRoutine : Inport  Port=3
  sensorView : Inport  Port=4
  targetReached : Inport  Port=5
  Action Port : ActionPort  ActionType=case
  Chart : Stateflow chart  TreatAsAtomicUnit=on
  Constant1 : Constant  Value=FORWARD
  Constant10 : Constant  Value=LEFT_EMPTY_RIGHT_BUSY
  Constant11 : Constant  Value=LEFT_EMPTY_RIGHT_CLEANED
  Constant12 : Constant  Value=LEFT_EMPTY_RIGHT_EMPTY
  Constant13 : Constant  Value=LEFT_BUSY_RIGHT_BUSY
  Constant14 : Constant  Value=LEFT_CLEANED_RIGHT_CLEANED
  Constant15 : Constant  Value=LEFT_BUSY_RIGHT_CLEANED
  Constant16 : Constant  Value=LEFT_CLEANED_RIGHT_BUSY
  Constant18 : Constant  Value=ROB_NORTH
  Constant19 : Constant  Value=ROB_SOUTH
  Constant2 : Constant  Value=MOVE_TURN_LEFT
  Constant20 : Constant  Value=ROB_WEST
  Constant21 : Constant  Value=ROB_EAST
  Constant3 : Constant  Value=MOVE_TURN_RIGHT
  Constant4 : Constant  Value=MOVE_U_TURN
  Constant5 : Constant  Value=MOVE_U_TURN_RIGHT
  Constant6 : Constant  Value=MOVE_U_TURN_LEFT
  Constant7 : Constant  Value=STOP
  Constant8 : Constant  Value=LEFT_BUSY_RIGHT_EMPTY
  Constant9 : Constant  Value=LEFT_CLEANED_RIGHT_EMPTY
  moveRequest : Outport
  zgzgActive : Outport  Port=2  InitialOutput=true
  wires:
  Constant21/1 -> Chart/13(ROB_EAST)
  Constant8/1 -> Chart/1(LEFT_BUSY_RIGHT_EMPTY)
  Constant9/1 -> Chart/2(LEFT_CLEANED_RIGHT_EMPTY)
  Constant20/1 -> Chart/12(ROB_WEST)
  Constant13/1 -> Chart/6(LEFT_BUSY_RIGHT_BUSY)
  Constant15/1 -> Chart/8(LEFT_BUSY_RIGHT_CLEANED)
  Constant18/1 -> Chart/10(ROB_NORTH)
  Constant19/1 -> Chart/11(ROB_SOUTH)
  Constant14/1 -> Chart/7(LEFT_CLEANED_RIGHT_CLEANED)
  Constant11/1 -> Chart/4(LEFT_EMPTY_RIGHT_CLEANED)
  Constant12/1 -> Chart/5(LEFT_EMPTY_RIGHT_EMPTY)
  Constant10/1 -> Chart/3(LEFT_EMPTY_RIGHT_BUSY)
  Constant16/1 -> Chart/9(LEFT_CLEANED_RIGHT_BUSY)
  Constant1/1 -> Chart/14(FORWARD)
  Constant4/1 -> Chart/17(MOVE_U_TURN)
  Constant3/1 -> Chart/16(MOVE_TURN_RIGHT)
  Constant2/1 -> Chart/15(MOVE_TURN_LEFT)
  Constant6/1 -> Chart/19(MOVE_U_TURN_LEFT)
  Constant5/1 -> Chart/18(MOVE_U_TURN_RIGHT)
  pumperInterrupt_BOOL/1 -> Chart/24(pumperInterrupt_BOOL)
  sensorView/1 -> Chart/20(sensorView)
  currentRoutine/1 -> Chart/23(currentRoutine)
  currentHeading/1 -> Chart/22(currentHeading)
  Constant7/1 -> Chart/21(STOP)
  Chart/1(moveRequest) -> moveRequest/1
  Chart/2(zgzgActive) -> zgzgActive/1
  targetReached/1 -> Chart/25(targetReached)

== system RobotControl/Compass_Handler/Subsystem1/OMEGA_Calc ==
  Vr : Inport
  Vl : Inport  Port=2
  Add : Sum  Inputs=+-
  Constant3 : Constant  Value=ROB_LENG
  Divide1 : Product  Inputs=*/
  W : Outport
  wires:
  Vl/1 -> Add/2
  Vr/1 -> Add/1
  Constant3/1 -> Divide1/2
  Divide1/1 -> W/1
  Add/1 -> Divide1/1

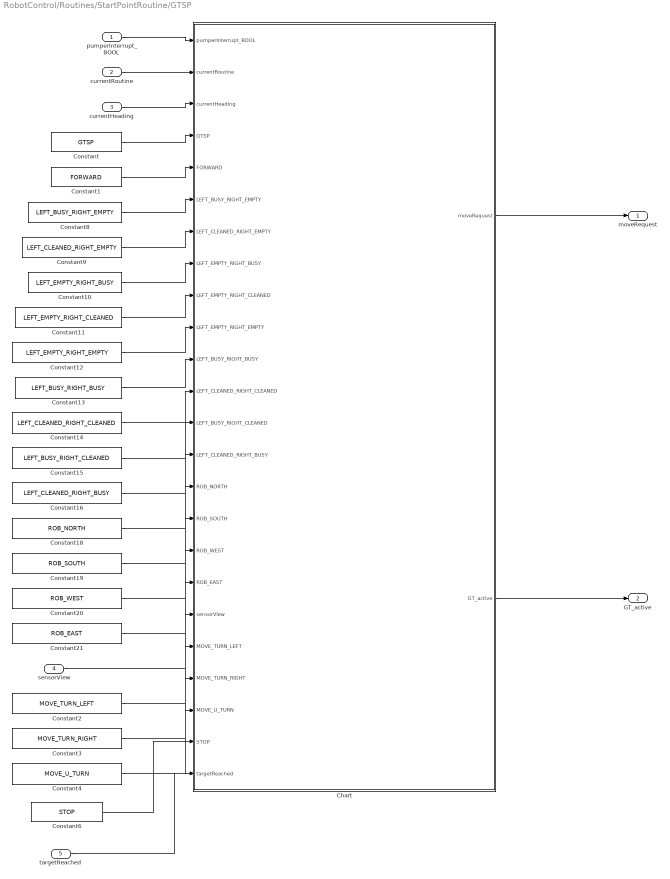
== system RobotControl/Routines/StartPointRoutine/GTSP ==
  pumperInterrupt_BOOL : Inport
  currentRoutine : Inport  Port=2
  currentHeading : Inport  Port=3
  sensorView : Inport  Port=4
  targetReached : Inport  Port=5
  Chart : Stateflow chart  TreatAsAtomicUnit=on
  Constant : Constant  Value=GTSP
  Constant1 : Constant  Value=FORWARD
  Constant10 : Constant  Value=LEFT_EMPTY_RIGHT_BUSY
  Constant11 : Constant  Value=LEFT_EMPTY_RIGHT_CLEANED
  Constant12 : Constant  Value=LEFT_EMPTY_RIGHT_EMPTY
  Constant13 : Constant  Value=LEFT_BUSY_RIGHT_BUSY
  Constant14 : Constant  Value=LEFT_CLEANED_RIGHT_CLEANED
  Constant15 : Constant  Value=LEFT_BUSY_RIGHT_CLEANED
  Constant16 : Constant  Value=LEFT_CLEANED_RIGHT_BUSY
  Constant18 : Constant  Value=ROB_NORTH
  Constant19 : Constant  Value=ROB_SOUTH
  Constant2 : Constant  Value=MOVE_TURN_LEFT
  Constant20 : Constant  Value=ROB_WEST
  Constant21 : Constant  Value=ROB_EAST
  Constant3 : Constant  Value=MOVE_TURN_RIGHT
  Constant4 : Constant  Value=MOVE_U_TURN
  Constant6 : Constant  Value=STOP
  Constant8 : Constant  Value=LEFT_BUSY_RIGHT_EMPTY
  Constant9 : Constant  Value=LEFT_CLEANED_RIGHT_EMPTY
  moveRequest : Outport
  GT_active : Outport  Port=2
  wires:
  Constant6/1 -> Chart/23(STOP)
  Chart/2(GT_active) -> GT_active/1
  Chart/1(moveRequest) -> moveRequest/1
  Constant2/1 -> Chart/20(MOVE_TURN_LEFT)
  Constant3/1 -> Chart/21(MOVE_TURN_RIGHT)
  Constant4/1 -> Chart/22(MOVE_U_TURN)
  sensorView/1 -> Chart/19(sensorView)
  Constant18/1 -> Chart/15(ROB_NORTH)
  Constant19/1 -> Chart/16(ROB_SOUTH)
  Constant20/1 -> Chart/17(ROB_WEST)
  Constant21/1 -> Chart/18(ROB_EAST)
  Constant16/1 -> Chart/14(LEFT_CLEANED_RIGHT_BUSY)
  Constant15/1 -> Chart/13(LEFT_BUSY_RIGHT_CLEANED)
  Constant14/1 -> Chart/12(LEFT_CLEANED_RIGHT_CLEANED)
  Constant13/1 -> Chart/11(LEFT_BUSY_RIGHT_BUSY)
  Constant12/1 -> Chart/10(LEFT_EMPTY_RIGHT_EMPTY)
  Constant11/1 -> Chart/9(LEFT_EMPTY_RIGHT_CLEANED)
  Constant10/1 -> Chart/8(LEFT_EMPTY_RIGHT_BUSY)
  Constant9/1 -> Chart/7(LEFT_CLEANED_RIGHT_EMPTY)
  Constant8/1 -> Chart/6(LEFT_BUSY_RIGHT_EMPTY)
  Constant1/1 -> Chart/5(FORWARD)
  Constant/1 -> Chart/4(GTSP)
  currentRoutine/1 -> Chart/2(currentRoutine)
  pumperInterrupt_BOOL/1 -> Chart/1(pumperInterrupt_BOOL)
  currentHeading/1 -> Chart/3(currentHeading)
  targetReached/1 -> Chart/24(targetReached)

== stateflow chart RobotControl/Routines/StartPointRoutine/GTSP/Chart ==
  state Idle
    entry:
    counter = 0;
    moveRequest = STOP;
    du:
    counter++;
  state GTSP_Active
    state Forward
      entry:
      moveRequest = FORWARD;
    state TurnLeft
      entry:
      moveRequest = MOVE_TURN_LEFT;
    state preFinishLeftBlockedN
      entry:
      moveRequest = MOVE_U_TURN;
    state preFinishLeftBlockedW
      entry:
      moveRequest = MOVE_TURN_RIGHT;
    state preFinishNormal
      entry:
      moveRequest = MOVE_TURN_LEFT;
    state preFinishBlockedW
    state preFinishBlockedN
      entry:
      moveRequest = MOVE_U_TURN;
    state finishedGTSP
      entry:
      moveRequest = STOP;
      GT_active = false;
    TurnLeft -> Forward : [(currentHeading == ROB_WEST)...
        | && (targetReached == true)]
    (default) -> Forward
    Forward -> (junction 14) : [pumperInterrupt_BOOL]
        | /moveRequest = STOP;
    (junction 14) -> (junction 17) [order 1] : [(sensorView == LEFT_EMPTY_RIGHT_EMPTY)...
        | || (sensorView == LEFT_EMPTY_RIGHT_CLEANED)...
        | || (sensorView == LEFT_EMPTY_RIGHT_BUSY)]
    (junction 14) -> (junction 22) [order 2] : [(sensorView == LEFT_CLEANED_RIGHT_EMPTY)...
        | || (sensorView == LEFT_BUSY_RIGHT_EMPTY)]
    (junction 14) -> (junction 29) [order 3] : [(sensorView == LEFT_BUSY_RIGHT_BUSY)...
        | || (sensorView == LEFT_BUSY_RIGHT_CLEANED)...
        | || (sensorView == LEFT_CLEANED_RIGHT_BUSY)...
        | || (sensorView == LEFT_CLEANED_RIGHT_CLEANED)]
    (junction 17) -> TurnLeft [order 1] : [currentHeading == ROB_NORTH]
    (junction 17) -> preFinishNormal [order 2] : [currentHeading == ROB_WEST]
    (junction 22) -> preFinishLeftBlockedW [order 2] : [currentHeading == ROB_WEST]
    (junction 22) -> preFinishLeftBlockedN [order 1] : [currentHeading == ROB_NORTH]
    (junction 29) -> preFinishBlockedW [order 1] : [currentHeading == ROB_WEST]
    (junction 29) -> preFinishBlockedN [order 2] : [currentHeading == ROB_NORTH]
    preFinishLeftBlockedN -> finishedGTSP : [(currentHeading == ROB_SOUTH)...
        | && (targetReached == true)]
    preFinishLeftBlockedW -> finishedGTSP : [(currentHeading == ROB_NORTH)...
        | && (targetReached == true)]
    preFinishNormal -> finishedGTSP : [(currentHeading == ROB_SOUTH)...
        | && (targetReached == true)]
    preFinishBlockedN -> finishedGTSP : [(currentHeading == ROB_NORTH)...
        | && (targetReached == true)]
    preFinishBlockedW -> finishedGTSP
  (default) -> Idle
  Idle -> GTSP_Active : [(currentRoutine == GTSP)...
      | && (counter > 200)]
      | /GT_active = true;
  GTSP_Active -> Idle : [currentRoutine != GTSP]
  data: pumperInterrupt_BOOL input; currentRoutine input; currentHeading input; GTSP input; FORWARD input; LEFT_BUSY_RIGHT_EMPTY input; LEFT_CLEANED_RIGHT_EMPTY input; LEFT_EMPTY_RIGHT_BUSY input; LEFT_EMPTY_RIGHT_CLEANED input; LEFT_EMPTY_RIGHT_EMPTY input; LEFT_BUSY_RIGHT_BUSY input; LEFT_CLEANED_RIGHT_CLEANED input; LEFT_BUSY_RIGHT_CLEANED input; LEFT_CLEANED_RIGHT_BUSY input; ROB_NORTH input; ROB_SOUTH input; ROB_WEST input; ROB_EAST input; sensorView input; moveRequest output uint8; MOVE_TURN_LEFT input; MOVE_TURN_RIGHT input; MOVE_U_TURN input; GT_active output boolean =true; STOP input; targetReached input; counter local double

== stateflow chart RobotControl/MovementHandler/EncoderHandler/singleStepCalc ==
  state Running
    state PosEdge
      entry:
      counter++;
    state High
    state step
      entry:
      step = true;
      counter = 0;
    (default) -> High
    High -> PosEdge : [hasChanged(encoderTicks_BOOL)...
        | && encoderTicks_BOOL == true]
        | /step = false;
    PosEdge -> High [order 2]
    step -> High
    PosEdge -> step [order 1] : [counter >= 86]
  state Idle
    state Rise
      en:
      step = true;
    state Idle
      en:
      step = false;
    (default) -> (junction 23)
    (junction 23) -> Rise [order 1] : [counter >= (86*0.75)]
    (junction 23) -> Idle.Idle [order 2]
  state Init
    entry:
    counter = 0;
  (default) -> Init
  Init -> Running
  Running -> Idle : [EnableConditions == false]
      | /step = false;
  Idle -> Running : [EnableConditions == true]
      | /step = false;
      | counter = 0;
  data: encoderTicks_BOOL input; step output boolean; counter local uint8; EnableConditions input; stepOld input boolean

== stateflow chart RobotControl/MovementHandler/HighLevelMoves ==
  state Stop
  state forward
    state fixingHeading
    state Idle
    (junction 252) -> fixingHeading [order 1] : [(rawTheta < 90*100)...
        | || (rawTheta > 270*100)]
        | /turnRequest = CCW;
    (default) -> Idle
    (junction 252) -> fixingHeading [order 2] : /turnRequest = CW;
    (junction 250) -> (junction 252) [order 1] : [headingRequest == ROB_NORTH]
    (junction 253) -> fixingHeading [order 1] : [(rawTheta < 90*100)...
        | || (rawTheta > 270*100)]
        | /turnRequest = CW;
    (junction 250) -> (junction 253) [order 2] : [headingRequest == ROB_SOUTH]
    (junction 253) -> fixingHeading [order 2] : /turnRequest = CCW;
    Idle -> (junction 270)
    (junction 270) -> (junction 250) [order 1] : [!((rawTheta >= (headingRequest*100) - 300)...
        | && (rawTheta <= (headingRequest*100) + 300))]
    (junction 250) -> (junction 254) [order 3] : [headingRequest == ROB_EAST]
    (junction 270) -> Idle [order 2] : [(rawTheta >= (headingRequest*100) - 300)...
        | && (rawTheta <= (headingRequest*100) + 300)]
        | /turnRequest = FORWARD;
    (junction 250) -> (junction 255) [order 4] : [headingRequest == ROB_WEST]
    (junction 254) -> fixingHeading [order 1] : [rawTheta > 180*100]
        | /turnRequest = CW;
    (junction 254) -> fixingHeading [order 2] : /turnRequest = CCW;
    (junction 255) -> fixingHeading [order 1] : [rawTheta > 180*100]
        | /turnRequest = CCW;
    fixingHeading -> Idle
    (junction 255) -> fixingHeading [order 2] : /turnRequest = CW;
  state TurnLeft
    state finish
      entry:
      turnActive = false;
    state start
      entry:
      turnRequest = CCW;
      turnActive = true;
    state turning
    (default) -> TurnLeft.start
    TurnLeft.start -> TurnLeft.turning [order 1] : [currentHeading == ROB_NORTH]
        | /headingRequest = ROB_WEST;
    TurnLeft.start -> TurnLeft.turning [order 3] : [currentHeading == ROB_SOUTH]
        | /headingRequest = ROB_EAST;
    TurnLeft.turning -> TurnLeft.finish : [(currentHeading == headingRequest)...
        | && (targetReached == true)]
    TurnLeft.start -> TurnLeft.turning [order 4] : [currentHeading == ROB_WEST]
        | /headingRequest = ROB_SOUTH;
    TurnLeft.start -> TurnLeft.turning [order 2] : [currentHeading == ROB_EAST]
        | /headingRequest = ROB_NORTH;
  state backward
  state UturnLeft
    entry:
    uTurnCounter = 0;
    state finish
      entry:
      turnActive = false;
    state TurnLeft
      state finish
        entry:
        uTurnCounter = uTurnCounter + 1;
      state start
        entry:
        turnRequest = CCW;
        turnActive = true;
      state turning
      (default) -> UturnLeft.TurnLeft.start
      UturnLeft.TurnLeft.start -> UturnLeft.TurnLeft.turning [order 1] : [currentHeading == ROB_NORTH]
          | /headingRequest = ROB_WEST;
      UturnLeft.TurnLeft.start -> UturnLeft.TurnLeft.turning [order 3] : [currentHeading == ROB_SOUTH]
          | /headingRequest = ROB_EAST;
      UturnLeft.TurnLeft.turning -> UturnLeft.TurnLeft.finish : [(currentHeading == headingRequest)...
          | && (targetReached == true)]
      UturnLeft.TurnLeft.start -> UturnLeft.TurnLeft.turning [order 4] : [currentHeading == ROB_WEST]
          | /headingRequest = ROB_SOUTH;
      UturnLeft.TurnLeft.start -> UturnLeft.TurnLeft.turning [order 2] : [currentHeading == ROB_EAST]
          | /headingRequest = ROB_NORTH;
    state forwardStep
      entry:
      counter = 0;
      turnRequest = FORWARD;
      currentMove = FORWARD;
      du:
      counter++;
    (default) -> UturnLeft.TurnLeft
    UturnLeft.TurnLeft -> UturnLeft.finish [order 2] : [uTurnCounter == 2]
    UturnLeft.TurnLeft -> UturnLeft.forwardStep [order 1] : [(uTurnCounter == 1)...
        | && hasChanged(uTurnCounter)]
    UturnLeft.forwardStep -> UturnLeft.TurnLeft [order 1] : [(counter >= 2)...
        | && moveDone == true]
        | /moveDone = false;
        | currentMove = MOVE_U_TURN_LEFT;
    UturnLeft.forwardStep -> UturnLeft.forwardStep [order 2] : [(hasChanged(completeStep))...
        | && (completeStep == true)]
        | /moveDone = true;
  state Uturn
    entry:
    uTurnCounter = 0;
    state finish
      entry:
      turnActive = false;
    state TurnRight
      state finish
        uTurnCounter = uTurnCounter + 1;
      state turning
      state start
        entry:
        turnRequest = CW;
        turnActive = true;
      (default) -> Uturn.TurnRight.start
      Uturn.TurnRight.start -> Uturn.TurnRight.turning [order 2] : [currentHeading == ROB_NORTH]
          | /headingRequest = ROB_EAST;
      Uturn.TurnRight.start -> Uturn.TurnRight.turning [order 4] : [currentHeading == ROB_SOUTH]
          | /headingRequest = ROB_WEST;
      Uturn.TurnRight.turning -> Uturn.TurnRight.finish : [(currentHeading == headingRequest)...
          | && (targetReached == true)]
      Uturn.TurnRight.start -> Uturn.TurnRight.turning [order 3] : [currentHeading == ROB_WEST]
          | /headingRequest = ROB_NORTH;
      Uturn.TurnRight.start -> Uturn.TurnRight.turning [order 1] : [currentHeading == ROB_EAST]
          | /headingRequest = ROB_SOUTH;
    Uturn.TurnRight -> Uturn.TurnRight [order 1] : [(uTurnCounter == 1)...
        | && hasChanged(uTurnCounter)]
    (default) -> Uturn.TurnRight
    Uturn.TurnRight -> Uturn.finish [order 2] : [uTurnCounter == 2]
  state TurnRight
    state turning
    state finish
      entry:
      turnActive = false;
    state start
      entry:
      turnRequest = CW;
      turnActive = true;
    (default) -> TurnRight.start
    TurnRight.start -> TurnRight.turning [order 2] : [currentHeading == ROB_NORTH]
        | /headingRequest = ROB_EAST;
    TurnRight.start -> TurnRight.turning [order 4] : [currentHeading == ROB_SOUTH]
        | /headingRequest = ROB_WEST;
    TurnRight.turning -> TurnRight.finish : [(currentHeading == headingRequest)...
        | && (targetReached == true)]
    TurnRight.start -> TurnRight.turning [order 3] : [currentHeading == ROB_WEST]
        | /headingRequest = ROB_NORTH;
    TurnRight.start -> TurnRight.turning [order 1] : [currentHeading == ROB_EAST]
        | /headingRequest = ROB_SOUTH;
  state UturnRight
    entry:
    uTurnCounter = 0;
    state finish
      entry:
      turnActive = false;
    state TurnRight
      state start
        entry:
        turnRequest = CW;
        turnActive = true;
      state finish
        entry:
        uTurnCounter = uTurnCounter + 1;
      state turning
      (default) -> UturnRight.TurnRight.start
      UturnRight.TurnRight.start -> UturnRight.TurnRight.turning [order 2] : [currentHeading == ROB_NORTH]
          | /headingRequest = ROB_EAST;
      UturnRight.TurnRight.start -> UturnRight.TurnRight.turning [order 4] : [currentHeading == ROB_SOUTH]
          | /headingRequest = ROB_WEST;
      UturnRight.TurnRight.turning -> UturnRight.TurnRight.finish : [(currentHeading...
          |  == headingRequest)...
          | && (targetReached == true)]
      UturnRight.TurnRight.start -> UturnRight.TurnRight.turning [order 3] : [currentHeading == ROB_WEST]
          | /headingRequest = ROB_NORTH;
      UturnRight.TurnRight.start -> UturnRight.TurnRight.turning [order 1] : [currentHeading == ROB_EAST]
          | /headingRequest = ROB_SOUTH;
    state forwardStep
      entry:
      counter = 0;
      turnRequest = FORWARD;
      currentMove = FORWARD;
      du:
      counter++;
    (default) -> UturnRight.TurnRight
    UturnRight.TurnRight -> UturnRight.finish [order 2] : [uTurnCounter == 2]
    UturnRight.TurnRight -> UturnRight.forwardStep [order 1] : [hasChanged(uTurnCounter) ...
        | && (uTurnCounter == 1)]
    UturnRight.forwardStep -> UturnRight.TurnRight [order 1] : [(counter >= 2)...
        | && moveDone == true]
        | /moveDone = false;
        | currentMove = MOVE_U_TURN_RIGHT;
    UturnRight.forwardStep -> UturnRight.forwardStep [order 2] : [(hasChanged(completeStep))...
        | && (completeStep == true)]
        | /moveDone = true;
  (default) -> Stop : /headingRequest = ROB_NORTH;
  Stop -> (junction 9) : [hasChanged(moveRequest) ...
      | || (turnActive == false)]
  (junction 9) -> Stop [order 6] : [moveRequest == STOP]
      | /turnRequest = STOP;
      | currentMove = STOP;
  forward -> (junction 9) : [hasChanged(moveRequest)]
  (junction 9) -> TurnLeft [order 8] : [(moveRequest == MOVE_TURN_LEFT)]
      | /currentMove = MOVE_TURN_LEFT;
  (junction 9) -> forward [order 1] : [moveRequest == FORWARD]
      | /turnRequest = FORWARD;
      | currentMove = FORWARD;
  TurnLeft -> (junction 9) : [hasChanged(moveRequest) ...
      | || (turnActive == false)]
  (junction 9) -> backward [order 2] : [moveRequest == BACKWARD]
      | /turnRequest = BACKWARD;
      | currentMove = BACKWARD;
  (junction 9) -> UturnLeft [order 5] : [(moveRequest == MOVE_U_TURN_LEFT)]
      | /currentMove = MOVE_U_TURN_LEFT;
  backward -> (junction 9) : [hasChanged(moveRequest) ...
      | || (turnActive == false)]
  Uturn -> (junction 9) : [hasChanged(moveRequest) ...
      | || (turnActive == false)]
  UturnLeft -> (junction 9) : [hasChanged(moveRequest) ...
      | || (turnActive == false)]
  (junction 9) -> TurnRight [order 7] : [(moveRequest == MOVE_TURN_RIGHT)]
      | /currentMove = MOVE_TURN_RIGHT;
  (junction 9) -> Uturn [order 4] : [moveRequest == MOVE_U_TURN]
      | /currentMove = MOVE_U_TURN;
  UturnRight -> (junction 9) : [hasChanged(moveRequest) ...
      | || (turnActive == false)]
  TurnRight -> (junction 9) : [hasChanged(moveRequest) ...
      | || (turnActive == false)]
  (junction 9) -> UturnRight [order 3] : [(moveRequest == MOVE_U_TURN_RIGHT)]
      | /currentMove = MOVE_U_TURN_RIGHT;
  data: moveRequest input; currentHeading input; FORWARD input; BACKWARD input; STOP input; MOVE_TURN_LEFT input; MOVE_TURN_RIGHT input; MOVE_U_TURN_LEFT input; MOVE_U_TURN_RIGHT input; MOVE_U_TURN input; turnRequest output double; headingRequest output double; CCW input double; CW input double; ROB_NORTH input; ROB_SOUTH input; ROB_WEST input; ROB_EAST input; rawTheta input; turnActive local double; completeStep input; uTurnCounter local double; currentX input; ROOM_SIDE_SIZE input; currentY input; counter local double; moveDone local double; currentMove output double; targetReached input
